simulink model "Enabled_Subsystem_Ex"  (R2021b)
settings: Solver=VariableStepAuto  StartTime=0.0  StopTime=10.0  RelTol=1e-3
settings Model: Creator=t  LastModifiedBy=t

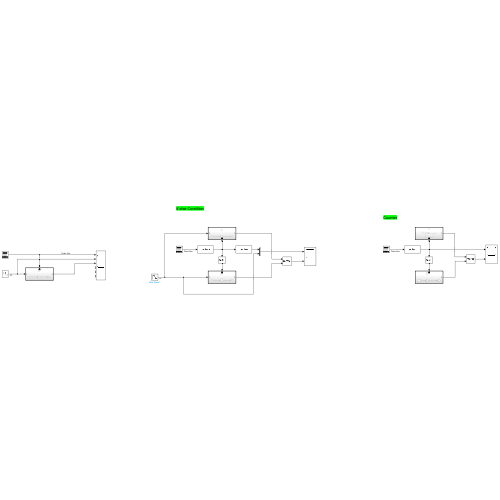
[thumbnail: Simulink's stored preview of the top-level diagram]
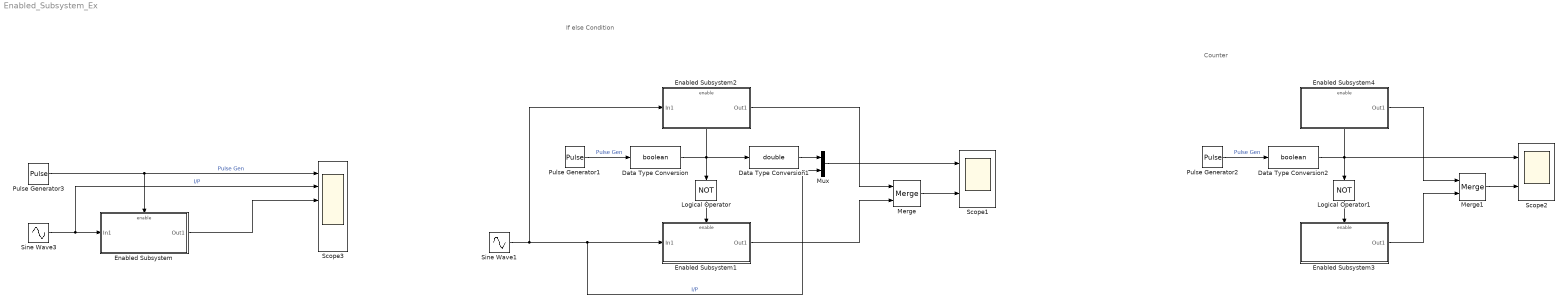
== system Enabled_Subsystem_Ex ==
  note: If else Condition
  note: Counter
  Data Type Conversion : DataTypeConversion  OutDataTypeStr=boolean
  Data Type Conversion1 : DataTypeConversion  OutDataTypeStr=double
  Data Type Conversion2 : DataTypeConversion  OutDataTypeStr=boolean
  Enabled Subsystem : Subsystem  TreatAsAtomicUnit=on
  Enabled Subsystem1 : Subsystem  TreatAsAtomicUnit=on
  Enabled Subsystem2 : Subsystem  TreatAsAtomicUnit=on
  Enabled Subsystem3 : Subsystem  TreatAsAtomicUnit=on
  Enabled Subsystem4 : Subsystem  TreatAsAtomicUnit=on
  Logical Operator : Logic  Operator=NOT  AllPortsSameDT=off  OutDataTypeStr=boolean
  Logical Operator1 : Logic  Operator=NOT  AllPortsSameDT=off  OutDataTypeStr=boolean
  Merge : Merge
  Merge1 : Merge
  Mux : Mux  Inputs=2
  Pulse Generator1 : DiscretePulseGenerator  Period=10  PulseWidth=5  SampleTime=0.2
  Pulse Generator2 : DiscretePulseGenerator  Period=10  PulseWidth=5  SampleTime=0.2
  Pulse Generator3 : DiscretePulseGenerator  Period=10  PulseWidth=5  SampleTime=0.2
  Scope1 : Scope  NumInputPorts=2
  Scope2 : Scope  NumInputPorts=2
  Scope3 : Scope  NumInputPorts=6
  Sine Wave1 : Sin  SampleTime=0.1
  Sine Wave3 : Sin  SampleTime=0.1
  wires:
  Sine Wave3/1 -> Scope3/2, Enabled Subsystem/1(In1)  "I/P"
  Pulse Generator3/1 -> Enabled Subsystem/Enable, Scope3/1  "Pulse Gen"
  Enabled Subsystem/1(Out1) -> Scope3/3
  Logical Operator/1 -> Enabled Subsystem1/Enable
  Pulse Generator1/1 -> Data Type Conversion/1  "Pulse Gen"
  Data Type Conversion/1 -> Enabled Subsystem2/Enable, Data Type Conversion1/1, Logical Operator/1
  Sine Wave1/1 -> Enabled Subsystem2/1(In1), Mux/2, Enabled Subsystem1/1(In1)  "I/P"
  Enabled Subsystem2/1(Out1) -> Merge/1
  Enabled Subsystem1/1(Out1) -> Merge/2
  Mux/1 -> Scope1/1
  Data Type Conversion1/1 -> Mux/1
  Merge/1 -> Scope1/2
  Merge1/1 -> Scope2/2
  Data Type Conversion2/1 -> Scope2/1, Logical Operator1/1, Enabled Subsystem4/Enable
  Enabled Subsystem3/1(Out1) -> Merge1/2
  Enabled Subsystem4/1(Out1) -> Merge1/1
  Pulse Generator2/1 -> Data Type Conversion2/1  "Pulse Gen"
  Logical Operator1/1 -> Enabled Subsystem3/Enable

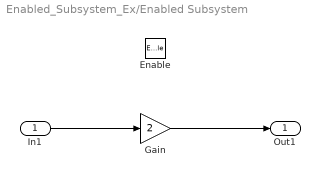
== system Enabled_Subsystem_Ex/Enabled Subsystem ==
  In1 : Inport
  Enable : EnablePort
  Gain : Gain  Gain=2
  Out1 : Outport
  wires:
  In1/1 -> Gain/1
  Gain/1 -> Out1/1

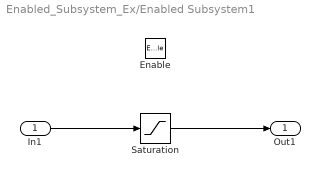
== system Enabled_Subsystem_Ex/Enabled Subsystem1 ==
  In1 : Inport
  Enable : EnablePort
  Saturation : Saturate  UpperLimit=0.75  LowerLimit=-0.75
  Out1 : Outport
  wires:
  Saturation/1 -> Out1/1
  In1/1 -> Saturation/1

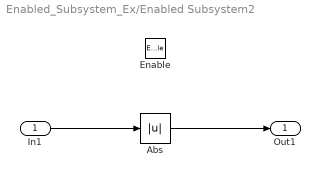
== system Enabled_Subsystem_Ex/Enabled Subsystem2 ==
  In1 : Inport
  Enable : EnablePort
  Abs : Abs
  Out1 : Outport
  wires:
  In1/1 -> Abs/1
  Abs/1 -> Out1/1

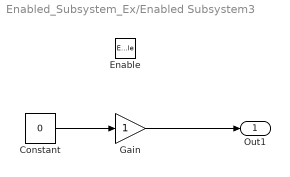
== system Enabled_Subsystem_Ex/Enabled Subsystem3 ==
  Enable : EnablePort
  Constant : Constant  Value=0
  Gain : Gain
  Out1 : Outport
  wires:
  Constant/1 -> Gain/1
  Gain/1 -> Out1/1

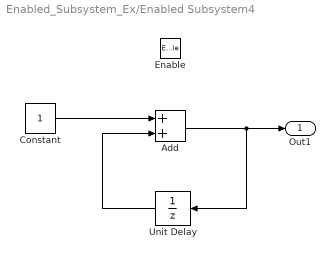
== system Enabled_Subsystem_Ex/Enabled Subsystem4 ==
  Enable : EnablePort
  Add : Sum
  Constant : Constant
  Unit Delay : UnitDelay  SampleTime=-1  HasFrameUpgradeWarning=on
  Out1 : Outport
  wires:
  Add/1 -> Unit Delay/1, Out1/1
  Constant/1 -> Add/1
  Unit Delay/1 -> Add/2
